simulink model "quadcopter"  (R2024a)
settings: Solver=VariableStepAuto  StartTime=0.0  StopTime=100  RelTol=1e-3
libraries: slpidlib x3
settings Model: Creator=ADMIN  LastModifiedBy=ADMIN

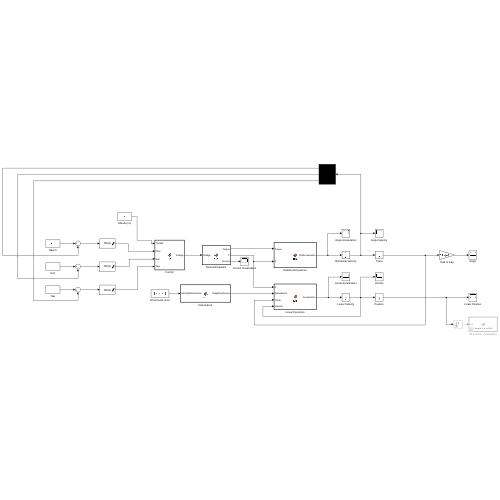
[thumbnail: Simulink's stored preview of the top-level diagram]
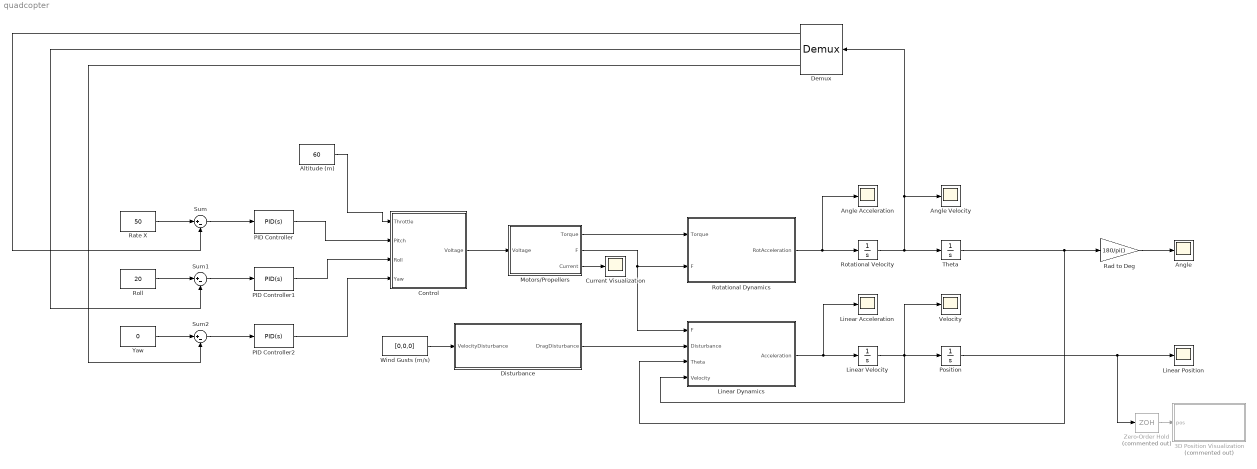
== system quadcopter ==
  3D Position Visualization : MATLAB Function  Commented=on  TreatAsAtomicUnit=on
  Altitude (m) : Constant  Value=60
  Angle : Scope
  Angle Acceleration : Scope
  Angle Velocity : Scope
  Control : MATLAB Function  TreatAsAtomicUnit=on
  Current Visualization : Scope
  Demux : Demux  Outputs=3
  Disturbance : MATLAB Function  TreatAsAtomicUnit=on
  Linear Acceleration : Scope
  Linear Dynamics : MATLAB Function  TreatAsAtomicUnit=on
  Linear Position : Scope
  Linear Velocity : Integrator
  Motors/Propellers : MATLAB Function  TreatAsAtomicUnit=on
  PID Controller : slpidlib/PID Controller  Controller=PID  Form=Parallel  TimeDomain=Continuous-time  UseExternalTs=off  SampleTime=-1  IntegratorMethod=Forward Euler  FilterMethod=Forward Euler  ControllerParametersSource=internal  P=10  I=5  UseKiTs=off  D=0  UseExternalDerivativeSource=off  N=100  UseFilter=on  TunerSelectOption=Transfer Function Based (PID Tuner App)  InitialConditionSource=internal  InitialConditionForIntegrator=0  InitialConditionForFilter=0  DifferentiatorICPrevScaledInput=0  ExternalReset=none  TrackingMode=off  Kt=1  LimitOutput=on  SatLimitsSource=internal  UpperSaturationLimit=100  LowerSaturationLimit=0  LinearizeAsGain=on  AntiWindupMode=clamping  Kb=1  LimitIntegrator=off  UpperIntegratorSaturationLimit=inf  LowerIntegratorSaturationLimit=-inf  POutMin=[]  POutMax=[]  IOutMin=[]  IOutMax=[]  DOutMin=[]  DOutMax=[]  NOutMin=[]  NOutMax=[]  SumOutMin=[]  SumOutMax=[]  SaturationOutMin=[]  SaturationOutMax=[]  PParamMin=[]  PParamMax=[]  IParamMin=[]  IParamMax=[]  DParamMin=[]  DParamMax=[]  NParamMin=[]  NParamMax=[]  KbParamMin=[]  KbParamMax=[]  KtParamMin=[]  KtParamMax=[]  KbOutMin=[]  KbOutMax=[]  KtOutMin=[]  KtOutMax=[]  IntegratorOutMin=[]  IntegratorOutMax=[]  FilterOutMin=[]  FilterOutMax=[]  SumI1OutMin=[]  SumI1OutMax=[]  SumI2OutMin=[]  SumI2OutMax=[]  SumI3OutMin=[]  SumI3OutMax=[]  SumI4OutMin=[]  SumI4OutMax=[]  SumDOutMin=[]  SumDOutMax=[]  DifferentiatorOutMin=[]  DifferentiatorOutMax=[]  FilterDiffOutCoefMin=[]  FilterDiffOutCoefMax=[]  ReciprocalOutMin=[]  ReciprocalOutMax=[]  SumDenOutMin=[]  SumDenOutMax=[]  SumNumOutMin=[]  SumNumOutMax=[]  DivideOutMin=[]  DivideOutMax=[]  UdiffTsProdOutMin=[]  UdiffTsProdOutMax=[]  NTsProdOutMin=[]  NTsProdOutMax=[]  UintegralTsProdOutMin=[]  UintegralTsProdOutMax=[]  UngainTsProdOutMin=[]  UngainTsProdOutMax=[]  ClampingZeroOutDataTypeStr=Inherit: Inherit via back propagation  ClampingZeroOutMin=[]  ClampingZeroOutMax=[]  FilterDenConstantOutDataTypeStr=Inherit: Inherit via back propagation  FilterDenConstantOutMin=[]  FilterDenConstantOutMax=[]  PCopyOutDataTypeStr=Inherit: Inherit via back propagation  PCopyOutMin=[]  PCopyOutMax=[]  NCopyOutDataTypeStr=Inherit: Inherit via back propagation  NCopyOutMin=[]  NCopyOutMax=[]  IntegratorContinuousStateAttributes=''  IntegratorStateMustResolveToSignalObject=off  IntegratorRTWStateStorageClass=Auto  FilterContinuousStateAttributes=''  FilterStateMustResolveToSignalObject=off  FilterRTWStateStorageClass=Auto  ParallelPVariant=InternalParameters  IdealPVariant=Disabled  IVariant=InternalParameters  DVariant=InternalParameters  IntegratorVariant=Continuous  SatVariant=Enabled  AWVariant=ContClampingParallel  PCopyVariant=Disabled  TRVariant=Disabled  FdbkBlocksVariant=Forward  IdealPFdbkVariant=Disabled  SatFdbkVariant=Disabled  DerivativeFilterVariant=ContFilter  NVariant=InternalParameters  NCopyVariant=Disabled  FilterICVariant=InternalICsFilter  IntegratorICVariant=InternalICs  ExternalResetVariant=Disabled  TRSumVariant=Passthrough  SumFdbkVariant=Disabled  SumVariant=Sum_PID  TsampFilterVariant=InternalTs  TsampNgainVariant=Passthrough  TsampIntegralVariant=Disabled_SignalSpec  ExternalSaturationOutDataTypeStr=Inherit: Same as second input  DerivativeSourceVariant=ErrorSignal
  PID Controller1 : slpidlib/PID Controller  Controller=PID  Form=Parallel  TimeDomain=Continuous-time  UseExternalTs=off  SampleTime=-1  IntegratorMethod=Forward Euler  FilterMethod=Forward Euler  ControllerParametersSource=internal  P=10  I=5  UseKiTs=off  D=0  UseExternalDerivativeSource=off  N=100  UseFilter=on  TunerSelectOption=Transfer Function Based (PID Tuner App)  InitialConditionSource=internal  InitialConditionForIntegrator=0  InitialConditionForFilter=0  DifferentiatorICPrevScaledInput=0  ExternalReset=none  TrackingMode=off  Kt=1  LimitOutput=on  SatLimitsSource=internal  UpperSaturationLimit=100  LowerSaturationLimit=0  LinearizeAsGain=on  AntiWindupMode=clamping  Kb=1  LimitIntegrator=off  UpperIntegratorSaturationLimit=inf  LowerIntegratorSaturationLimit=-inf  POutMin=[]  POutMax=[]  IOutMin=[]  IOutMax=[]  DOutMin=[]  DOutMax=[]  NOutMin=[]  NOutMax=[]  SumOutMin=[]  SumOutMax=[]  SaturationOutMin=[]  SaturationOutMax=[]  PParamMin=[]  PParamMax=[]  IParamMin=[]  IParamMax=[]  DParamMin=[]  DParamMax=[]  NParamMin=[]  NParamMax=[]  KbParamMin=[]  KbParamMax=[]  KtParamMin=[]  KtParamMax=[]  KbOutMin=[]  KbOutMax=[]  KtOutMin=[]  KtOutMax=[]  IntegratorOutMin=[]  IntegratorOutMax=[]  FilterOutMin=[]  FilterOutMax=[]  SumI1OutMin=[]  SumI1OutMax=[]  SumI2OutMin=[]  SumI2OutMax=[]  SumI3OutMin=[]  SumI3OutMax=[]  SumI4OutMin=[]  SumI4OutMax=[]  SumDOutMin=[]  SumDOutMax=[]  DifferentiatorOutMin=[]  DifferentiatorOutMax=[]  FilterDiffOutCoefMin=[]  FilterDiffOutCoefMax=[]  ReciprocalOutMin=[]  ReciprocalOutMax=[]  SumDenOutMin=[]  SumDenOutMax=[]  SumNumOutMin=[]  SumNumOutMax=[]  DivideOutMin=[]  DivideOutMax=[]  UdiffTsProdOutMin=[]  UdiffTsProdOutMax=[]  NTsProdOutMin=[]  NTsProdOutMax=[]  UintegralTsProdOutMin=[]  UintegralTsProdOutMax=[]  UngainTsProdOutMin=[]  UngainTsProdOutMax=[]  ClampingZeroOutDataTypeStr=Inherit: Inherit via back propagation  ClampingZeroOutMin=[]  ClampingZeroOutMax=[]  FilterDenConstantOutDataTypeStr=Inherit: Inherit via back propagation  FilterDenConstantOutMin=[]  FilterDenConstantOutMax=[]  PCopyOutDataTypeStr=Inherit: Inherit via back propagation  PCopyOutMin=[]  PCopyOutMax=[]  NCopyOutDataTypeStr=Inherit: Inherit via back propagation  NCopyOutMin=[]  NCopyOutMax=[]  IntegratorContinuousStateAttributes=''  IntegratorStateMustResolveToSignalObject=off  IntegratorRTWStateStorageClass=Auto  FilterContinuousStateAttributes=''  FilterStateMustResolveToSignalObject=off  FilterRTWStateStorageClass=Auto  ParallelPVariant=InternalParameters  IdealPVariant=Disabled  IVariant=InternalParameters  DVariant=InternalParameters  IntegratorVariant=Continuous  SatVariant=Enabled  AWVariant=ContClampingParallel  PCopyVariant=Disabled  TRVariant=Disabled  FdbkBlocksVariant=Forward  IdealPFdbkVariant=Disabled  SatFdbkVariant=Disabled  DerivativeFilterVariant=ContFilter  NVariant=InternalParameters  NCopyVariant=Disabled  FilterICVariant=InternalICsFilter  IntegratorICVariant=InternalICs  ExternalResetVariant=Disabled  TRSumVariant=Passthrough  SumFdbkVariant=Disabled  SumVariant=Sum_PID  TsampFilterVariant=InternalTs  TsampNgainVariant=Passthrough  TsampIntegralVariant=Disabled_SignalSpec  ExternalSaturationOutDataTypeStr=Inherit: Same as second input  DerivativeSourceVariant=ErrorSignal
  PID Controller2 : slpidlib/PID Controller  Controller=PID  Form=Parallel  TimeDomain=Continuous-time  UseExternalTs=off  SampleTime=-1  IntegratorMethod=Forward Euler  FilterMethod=Forward Euler  ControllerParametersSource=internal  P=10  I=5  UseKiTs=off  D=0  UseExternalDerivativeSource=off  N=100  UseFilter=on  TunerSelectOption=Transfer Function Based (PID Tuner App)  InitialConditionSource=internal  InitialConditionForIntegrator=0  InitialConditionForFilter=0  DifferentiatorICPrevScaledInput=0  ExternalReset=none  TrackingMode=off  Kt=1  LimitOutput=on  SatLimitsSource=internal  UpperSaturationLimit=100  LowerSaturationLimit=0  LinearizeAsGain=on  AntiWindupMode=clamping  Kb=1  LimitIntegrator=off  UpperIntegratorSaturationLimit=inf  LowerIntegratorSaturationLimit=-inf  POutMin=[]  POutMax=[]  IOutMin=[]  IOutMax=[]  DOutMin=[]  DOutMax=[]  NOutMin=[]  NOutMax=[]  SumOutMin=[]  SumOutMax=[]  SaturationOutMin=[]  SaturationOutMax=[]  PParamMin=[]  PParamMax=[]  IParamMin=[]  IParamMax=[]  DParamMin=[]  DParamMax=[]  NParamMin=[]  NParamMax=[]  KbParamMin=[]  KbParamMax=[]  KtParamMin=[]  KtParamMax=[]  KbOutMin=[]  KbOutMax=[]  KtOutMin=[]  KtOutMax=[]  IntegratorOutMin=[]  IntegratorOutMax=[]  FilterOutMin=[]  FilterOutMax=[]  SumI1OutMin=[]  SumI1OutMax=[]  SumI2OutMin=[]  SumI2OutMax=[]  SumI3OutMin=[]  SumI3OutMax=[]  SumI4OutMin=[]  SumI4OutMax=[]  SumDOutMin=[]  SumDOutMax=[]  DifferentiatorOutMin=[]  DifferentiatorOutMax=[]  FilterDiffOutCoefMin=[]  FilterDiffOutCoefMax=[]  ReciprocalOutMin=[]  ReciprocalOutMax=[]  SumDenOutMin=[]  SumDenOutMax=[]  SumNumOutMin=[]  SumNumOutMax=[]  DivideOutMin=[]  DivideOutMax=[]  UdiffTsProdOutMin=[]  UdiffTsProdOutMax=[]  NTsProdOutMin=[]  NTsProdOutMax=[]  UintegralTsProdOutMin=[]  UintegralTsProdOutMax=[]  UngainTsProdOutMin=[]  UngainTsProdOutMax=[]  ClampingZeroOutDataTypeStr=Inherit: Inherit via back propagation  ClampingZeroOutMin=[]  ClampingZeroOutMax=[]  FilterDenConstantOutDataTypeStr=Inherit: Inherit via back propagation  FilterDenConstantOutMin=[]  FilterDenConstantOutMax=[]  PCopyOutDataTypeStr=Inherit: Inherit via back propagation  PCopyOutMin=[]  PCopyOutMax=[]  NCopyOutDataTypeStr=Inherit: Inherit via back propagation  NCopyOutMin=[]  NCopyOutMax=[]  IntegratorContinuousStateAttributes=''  IntegratorStateMustResolveToSignalObject=off  IntegratorRTWStateStorageClass=Auto  FilterContinuousStateAttributes=''  FilterStateMustResolveToSignalObject=off  FilterRTWStateStorageClass=Auto  ParallelPVariant=InternalParameters  IdealPVariant=Disabled  IVariant=InternalParameters  DVariant=InternalParameters  IntegratorVariant=Continuous  SatVariant=Enabled  AWVariant=ContClampingParallel  PCopyVariant=Disabled  TRVariant=Disabled  FdbkBlocksVariant=Forward  IdealPFdbkVariant=Disabled  SatFdbkVariant=Disabled  DerivativeFilterVariant=ContFilter  NVariant=InternalParameters  NCopyVariant=Disabled  FilterICVariant=InternalICsFilter  IntegratorICVariant=InternalICs  ExternalResetVariant=Disabled  TRSumVariant=Passthrough  SumFdbkVariant=Disabled  SumVariant=Sum_PID  TsampFilterVariant=InternalTs  TsampNgainVariant=Passthrough  TsampIntegralVariant=Disabled_SignalSpec  ExternalSaturationOutDataTypeStr=Inherit: Same as second input  DerivativeSourceVariant=ErrorSignal
  Position : Integrator
  Rad to Deg : Gain  Gain=180/pi()
  Rate X : Constant  Value=50
  Roll : Constant  Value=20
  Rotational Dynamics : MATLAB Function  TreatAsAtomicUnit=on
  Rotational Velocity : Integrator
  Sum : Sum  Inputs=|+-
  Sum1 : Sum  Inputs=|+-
  Sum2 : Sum  Inputs=|+-
  Theta : Integrator
  Velocity : Scope
  Wind Gusts (m/s) : Constant  Value=[0,0,0]
  Yaw : Constant  Value=0
  Zero-Order Hold : ZeroOrderHold  Commented=on  SampleTime=0.001
  wires:
  Motors/Propellers/1(Torque) -> Rotational Dynamics/1(Torque)
  Motors/Propellers/2(F) -> Linear Dynamics/1(F), Rotational Dynamics/2(F)
  Rotational Dynamics/1(RotAcceleration) -> Angle Acceleration/1, Rotational Velocity/1
  Rotational Velocity/1 -> Demux/1, Angle Velocity/1, Theta/1
  Theta/1 -> Rad to Deg/1, Linear Dynamics/3(Theta)
  Linear Dynamics/1(Acceleration) -> Linear Acceleration/1, Linear Velocity/1
  Linear Velocity/1 -> Velocity/1, Linear Dynamics/4(Velocity), Position/1
  Disturbance/1(DragDisturbance) -> Linear Dynamics/2(Disturbance)
  Wind Gusts (m/s)/1 -> Disturbance/1(VelocityDisturbance)
  Control/1(Voltage) -> Motors/Propellers/1(Voltage)
  Position/1 -> Zero-Order Hold/1, Linear Position/1
  Rad to Deg/1 -> Angle/1
  Motors/Propellers/3(Current) -> Current Visualization/1
  Zero-Order Hold/1 -> 3D Position Visualization/1(pos)
  Rate X/1 -> Sum/1
  Sum/1 -> PID Controller/1
  Demux/1 -> Sum/2
  Altitude (m)/1 -> Control/1(Throttle)
  PID Controller/1 -> Control/2(Pitch)
  PID Controller1/1 -> Control/3(Roll)
  Demux/2 -> Sum1/2
  Roll/1 -> Sum1/1
  Sum1/1 -> PID Controller1/1
  PID Controller2/1 -> Control/4(Yaw)
  Yaw/1 -> Sum2/1
  Sum2/1 -> PID Controller2/1
  Demux/3 -> Sum2/2

== matlab function quadcopter/Rotational Dynamics ==
  data: Torque input; RotAcceleration output; F input
function RotAcceleration = fcn(Torque, F)
side_length = 0.237; % m

moment = [0 0 0]; % x y z
RotAcceleration = [0 0 0];
I = [0.003, 0.003, 0.007]; % kg.m2 - inertia

moment(1) = (F(3)+F(4))*side_length/2 - (F(1)+F(2))*side_length/2;
moment(2) = (F(3)+F(2))*side_length/2 - (F(1)+F(4))*side_length/2;
moment(3) = Torque(4) - Torque(1) + Torque(2) - Torque(3);

for i = 1:3
    RotAcceleration(i) = moment(i)/I(i);
end

== matlab function quadcopter/Motors//Propellers ==
  data: Voltage input; Torque output; F output; Current output
function [Torque, F, Current] = fcn(Voltage)
Kv  = 1400;   % RPM/V   - motor velocity constant
rho = 1.225;  % kg/m3   - air density 
D   = 0.2;    % m       - diameter of propeller

rpm     = [0 0 0 0];
Torque  = [0 0 0 0];
Current = [0 0 0 0];
F       = [0 0 0 0];

for i = 1:4
    rpm(i) = -2.6931*Voltage(i)^3 + Kv*Voltage(i);
    n = rpm(i)/60; % round per second
    Ct = 2*10^-15*rpm(i)^3 - 4*10^-11*rpm(i)^2 + 3*10^-7*rpm(i) + 0.1013;
    F(i) = Ct*rho*n^2*D^4;
    Torque(i) = 4*10^-14*rpm(i)^3 + 8*10^-12*rpm(i)^2 + 3*10^-6*rpm(i);
    Current(i) = Kv*Torque(i);
end

== matlab function quadcopter/Linear Dynamics ==
  data: F input; Disturbance input; Acceleration output; Theta input; Velocity input
function Acceleration = fcn(F, Disturbance, Theta, Velocity)
m = 0.743;
g = 9.81;
A = [0.0197 0.0197 0.0512]; % m2
rho = 1.225; % kg/m3 - air density
Cd = 1; % drag coef

Drag = [0 0 0];
for i = 1:3
    Drag(i) = 0.5*rho*Velocity(i)^2*A(i)*Cd;
end

Acceleration = [0 0 0];
Force = [0 0 0];
Fprop = [0 0 0];

Fprop(1) = sin(Theta(2))*cos(Theta(1))*(F(1)+F(2)+F(3)+F(4));
Fprop(2) = sin(Theta(1))*cos(Theta(2))*(F(1)+F(2)+F(3)+F(4));
Fprop(3) = cos(Theta(1))*cos(Theta(2))*(F(1)+F(2)+F(3)+F(4));

ThetaXY = -atan2(Fprop(1), Fprop(2));
XY2D = sqrt(Fprop(1)^2 + Fprop(2)^2);

if Fprop(3) >= 0
    Fprop(1) = XY2D*sin(ThetaXY+Theta(3));
    Fprop(2) = XY2D*cos(ThetaXY+Theta(3));
else
    Fprop(1) = XY2D*sin(ThetaXY-Theta(3));
    Fprop(2) = XY2D*cos(ThetaXY-Theta(3));
end

if Velocity(1) < 0
    Force(1) = Fprop(1) - Disturbance(1) + Drag(1);
else
    Force(1) = Fprop(1) - Disturbance(1) - Drag(1);
end

if Velocity(2) < 0
    Force(2) = Fprop(2) - Disturbance(2) + Drag(2);
else
    Force(2) = Fprop(2) - Disturbance(2) - Drag(2);
end

if Velocity(3) < 0
    Force(3) = Fprop(3) - Disturbance(3) + Drag(3) - m*g;
else
    Force(3) = Fprop(3) - Disturbance(3) - Drag(3) - m*g;
end

for i = 1:3
    Acceleration(i) = Force(i)/m;
end

== matlab function quadcopter/Disturbance ==
  data: VelocityDisturbance input; DragDisturbance output
function DragDisturbance = fcn(VelocityDisturbance)
A = [0.0197 0.0197 0.0197*2*1.3];
DragDisturbance = [0 0 0];
rho = 1.225;
Cd = 1;

for i = 1:3
    if VelocityDisturbance(i) < 0
        DragDisturbance(i) = 0.5*rho*VelocityDisturbance(i)^2*A(i)*Cd;
    else
        DragDisturbance(i) = -0.5*rho*VelocityDisturbance(i)^2*A(i)*Cd;
    end
end

== matlab function quadcopter/Control ==
  data: Throttle input; Voltage output; Pitch input; Roll input; Yaw input
function Voltage = fcn(Throttle, Pitch, Roll, Yaw)
Correct = 0;

if (Pitch/2+Roll/2+Yaw/2) > (100-Throttle)
    Correct = (Pitch/2+Roll/2+Yaw/2) - (100-Throttle);
end

if (Pitch/2+Roll/2+Yaw/2) > (Throttle)   % make sure the power never shut off
    if Correct < ((Pitch/2+Roll/2+Yaw/2) - (Throttle))
        Correct = (Pitch/2+Roll/2+Yaw/2) - (Throttle);
    end
end

if Correct ~= 0
    Pitch = Pitch - Correct/3*2;
    Roll = Roll - Correct/3*2;
    Yaw = Yaw - Correct/3*2;
end

Voltage = [(Throttle-Pitch/2-Roll/2-Yaw/2)*11.4/100     % altitude
           (Throttle-Pitch/2+Roll/2+Yaw/2)*11.4/100     % forward/backward
           (Throttle+Pitch/2+Roll/2-Yaw/2)*11.4/100     % right/left
           (Throttle+Pitch/2-Roll/2+Yaw/2)*11.4/100];   % yaw

== matlab function quadcopter/3D Position Visualization ==
  data: pos input
function visualize_position(pos)
    coder.extrinsic('plot3', 'drawnow', 'figure', 'isgraphics', 'gca', 'set', 'get', 'grid', 'xlabel', 'ylabel', 'zlabel');
    
    persistent fig hPlot
    
    if isempty(fig)
        fig = figure('Name', 'Live 3D Flight Path');
        
        % style
        hPlot = plot3(pos(1), pos(2), pos(3), 'b-', 'LineWidth', 1.5, ...
            'Marker', 'o', 'MarkerFaceColor', 'r', 'MarkerEdgeColor', 'k');
        
        grid('on');
        xlabel('X (m)'); 
        ylabel('Y (m)'); 
        zlabel('Altitude (m)');
        
        % set axes limit
        % set(gca, 'XLim', [-20 20], 'YLim', [-20 20], 'ZLim', [0 30]);
        axis('auto');
    end
    
    if isgraphics(fig)
        x_data = get(hPlot, 'XData');
        y_data = get(hPlot, 'YData');
        z_data = get(hPlot, 'ZData');
        
        new_X = [x_data, pos(1)];
        new_Y = [y_data, pos(2)];
        new_Z = [z_data, pos(3)];
        
        set(hPlot, 'XData', new_X, ...
                   'YData', new_Y, ...
                   'ZData', new_Z, ...
                   'MarkerIndices', length(new_X)); 
        
        drawnow limitrate;
    end
end
